simulink model "Getriebe_einfach"  (Simulink 7.1)
settings: Solver=ode45  StartTime=0.0  StopTime=10.0  RelTol=1e-3
undefined symbols (not defined in the file): i, Jc, Mlast
settings Model: Creator=dep19025415  LastModifiedBy=dep19025415

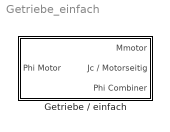
== system Getriebe_einfach ==
  Getriebe / einfach : Subsystem

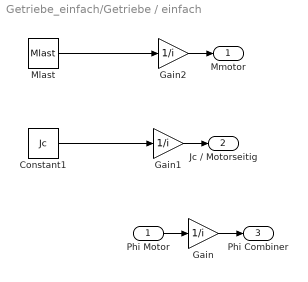
== system Getriebe_einfach/Getriebe / einfach ==
  Phi Motor : Inport
  Constant1 : Constant  Value=Jc  OutDataType=sfix(16)  OutScaling=2^0
  Gain : Gain  Gain=1/i  ParameterDataType=sfix(16)  ParameterScaling=2^0  OutDataType=sfix(16)  OutScaling=2^0
  Gain1 : Gain  Gain=1/i  ParameterDataType=sfix(16)  ParameterScaling=2^0  OutDataType=sfix(16)  OutScaling=2^0
  Gain2 : Gain  Gain=1/i  ParameterDataType=sfix(16)  ParameterScaling=2^0  OutDataType=sfix(16)  OutScaling=2^0
  Mlast : Constant  Value=Mlast  OutDataType=sfix(16)  OutScaling=2^0
  Mmotor : Outport
  Jc / Motorseitig : Outport  Port=2
  Phi Combiner : Outport  Port=3
  wires:
  Constant1/1 -> Gain1/1
  Mlast/1 -> Gain2/1
  Gain2/1 -> Mmotor/1
  Gain1/1 -> Jc / Motorseitig/1
  Phi Motor/1 -> Gain/1
  Gain/1 -> Phi Combiner/1
